simulink model "HANcoder_E407_GTSync_v3_clean"  (R2018b)
settings: Solver=FixedStepDiscrete  StartTime=0.0  StopTime=1  FixedStep=0.01  RelTol=1e-3
PreLoadFcn:
  | librarySetup
  | eval([bdroot,'_startup']) %Calling [modelName]_startup.m
values from neighbouring files (symbols this model uses):
  basic_cycle_duration = 60000    [HANcoder_E407_GTSync_v3_clean_startup.m]    (also in HANcoder_E407_GTSync_v3_startup.m = 50000)
  comm_delay_estimation = 3    [HANcoder_E407_GTSync_v3_clean_startup.m]
  frequency_IRQ = 100    [HANcoder_E407_GTSync_startup.m]    (also in HANcoder_E407_GTSync_v3_clean_startup.m = 99; HANcoder_E407_GTSync_v3_startup.m = 99)
  HANtuneOverride = Simulink.Parameter    [HANcoder_E407_GTSync_startup.m]    (also in HANcoder_E407_GTSync_v3_clean_startup.m; HANcoder_E407_GTSync_v3_startup.m)
  LED_ticks_toggle = 10000    [HANcoder_E407_GTSync_startup.m]    (also in HANcoder_E407_GTSync_v3_clean_startup.m; HANcoder_E407_GTSync_v3_startup.m)
  Master_Role = 1    [HANcoder_E407_GTSync_v3_clean_startup.m]    (also in HANcoder_E407_GTSync_v3_startup.m)
  matrix_rows = 2    [HANcoder_E407_GTSync_v3_clean_startup.m]    (also in HANcoder_E407_GTSync_v3_startup.m)
  Slave_Role = 2    [HANcoder_E407_GTSync_v3_clean_startup.m]    (also in HANcoder_E407_GTSync_v3_startup.m)
  Sync_ID = 1    [HANcoder_E407_GTSync_v3_clean_startup.m]    (also in HANcoder_E407_GTSync_v3_startup.m)
  time_difference_threshold = 500    [HANcoder_E407_GTSync_v3_clean_startup.m]    (also in HANcoder_E407_GTSync_v3_startup.m = 100)
  TM0 = 100    [HANcoder_E407_GTSync_v3_clean_startup.m]    (also in HANcoder_E407_GTSync_v3_startup.m = 0)
  TM1 = 20000    [HANcoder_E407_GTSync_v3_clean_startup.m]    (also in HANcoder_E407_GTSync_v3_startup.m = 25000)
  TM2 = 30000    [HANcoder_E407_GTSync_v3_clean_startup.m]    (also in HANcoder_E407_GTSync_v3_startup.m = 37500)
  TM3 = 40000    [HANcoder_E407_GTSync_v3_clean_startup.m]    (also in HANcoder_E407_GTSync_v3_startup.m)
  TM4 = 50000    [HANcoder_E407_GTSync_v3_clean_startup.m]
  Vote1_ID = 12    [HANcoder_E407_GTSync_v3_clean_startup.m]    (also in HANcoder_E407_GTSync_v3_startup.m)
  Vote2_ID = 22    [HANcoder_E407_GTSync_v3_clean_startup.m]    (also in HANcoder_E407_GTSync_v3_startup.m)
  Vote3_ID = 32    [HANcoder_E407_GTSync_v3_clean_startup.m]    (also in HANcoder_E407_GTSync_v3_startup.m)
  wrap_up_threshold = basic_cycle_duration - time_difference_threshold*10    (= 55000)    [HANcoder_E407_GTSync_v3_clean_startup.m]
libraries: HANcoder_STM32_Target x20, simulink x3, simulink_extras x1
(part 2 of 4)

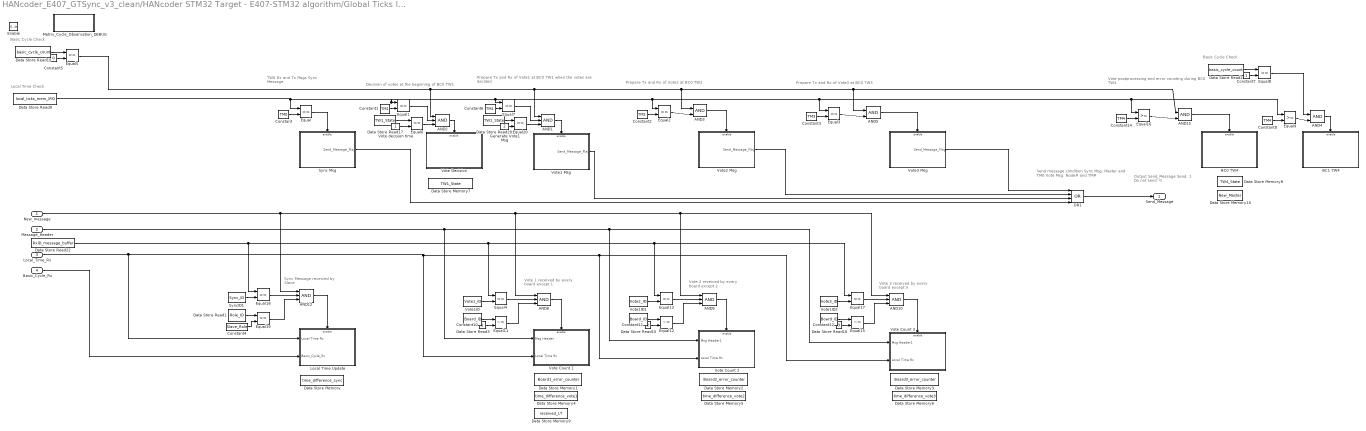
== system HANcoder_E407_GTSync_v3_clean/HANcoder STM32 Target - E407-STM32 algorithm/Global Ticks Increment/CAN Management/Matrix Cycle Manager ==
  note: Vote 3 received by
      | every board except 3
  note: Vote 2 received by
      | every board except 2
  note: Vote 1 received by
      | every board except 1
  note: Vote postprocessing and error
      | counting during BC0 TW4
  note: Prepare Tx and Rx of Vote3 at BC0 TW3
  note: Prepare Tx and Rx of Vote2 at BC0 TW2
  note: Prepare Tx and Rx of Vote1 at BC0 TW1
      | when the votes are decided
  note: Decision of votes at the beginning of BC0 TW1
  note: TW0 Rx and Tx Msgs
      | Sync Message
  note: Sync Message
      | received by Slave
  note: Local Time Check
  note: Output Send_Message
      | Send: 1
      | Do not send: 0
  note: Send message condition
      | Sync Msg: Master and TM0
      | Vote Msg: Node# and TM#
  note: Basic Cycle Check
  note: Basic Cycle Check
  New_message : Inport
  Message_Header : Inport  Port=2
  Local_Time_Rx : Inport  Port=3
  Basic_Cycle_Rx : Inport  Port=4
  Enable : EnablePort  PropagateVarSize=During execution
  AND{1..2,8..10,12} (6 alike) : Logic  Inputs=3  IconShape=distinctive  AllPortsSameDT=off  OutDataTypeStr=boolean
  AND{3..5,15} (4 alike) : Logic  IconShape=distinctive  AllPortsSameDT=off  OutDataTypeStr=boolean
  BC0 TW4 : Subsystem
  BC1 TW4 : Subsystem
  Constant : Constant  Value=TM0
  Constant1 : Constant  Value=TM1
  Constant10 : Constant
  Constant11 : Constant  Value=2
  Constant12 : Constant  Value=3
  Constant14 : Constant  Value=TM4
  Constant2 : Constant  Value=TM2
  Constant3 : Constant  Value=TM3
  Constant4 : Constant  Value=Slave_Role
  Constant5 : Constant  Value=0
  Constant6 : Constant  Value=TM1
  Constant7 : Constant
  Constant8 : Constant  Value=TM4
  Data Store Memory : DataStoreMemory  DataStoreName=time_difference_sync  ReadBeforeWriteMsg=warning  WriteAfterWriteMsg=warning  WriteAfterReadMsg=warning  ShowAdditionalParam=off
  Data Store Memory1 : DataStoreMemory  DataStoreName=Board1_error_counter  ReadBeforeWriteMsg=warning  WriteAfterWriteMsg=warning  WriteAfterReadMsg=warning  ShowAdditionalParam=off  OutMin=0  OutMax=4294967294  OutDataTypeStr=double
  Data Store Memory10 : DataStoreMemory  DataStoreName=New_Master  ReadBeforeWriteMsg=warning  WriteAfterWriteMsg=warning  WriteAfterReadMsg=warning  ShowAdditionalParam=off  OutDataTypeStr=boolean
  Data Store Memory2 : DataStoreMemory  DataStoreName=Board2_error_counter  ReadBeforeWriteMsg=warning  WriteAfterWriteMsg=warning  WriteAfterReadMsg=warning  ShowAdditionalParam=off  OutMin=0  OutMax=4294967294  OutDataTypeStr=double
  Data Store Memory3 : DataStoreMemory  DataStoreName=Board3_error_counter  ReadBeforeWriteMsg=warning  WriteAfterWriteMsg=warning  WriteAfterReadMsg=warning  ShowAdditionalParam=off  OutMin=0  OutMax=4294967294  OutDataTypeStr=double
  Data Store Memory4 : DataStoreMemory  DataStoreName=time_difference_vote1  ReadBeforeWriteMsg=warning  WriteAfterWriteMsg=warning  WriteAfterReadMsg=warning  ShowAdditionalParam=off
  Data Store Memory5 : DataStoreMemory  DataStoreName=time_difference_vote2  ReadBeforeWriteMsg=warning  WriteAfterWriteMsg=warning  WriteAfterReadMsg=warning  ShowAdditionalParam=off
  Data Store Memory6 : DataStoreMemory  DataStoreName=time_difference_vote3  ReadBeforeWriteMsg=warning  WriteAfterWriteMsg=warning  WriteAfterReadMsg=warning  ShowAdditionalParam=off
  Data Store Memory7 : DataStoreMemory  DataStoreName=TW1_State  ReadBeforeWriteMsg=warning  WriteAfterWriteMsg=warning  WriteAfterReadMsg=warning  InitialValue=1  ShowAdditionalParam=off
  Data Store Memory8 : DataStoreMemory  DataStoreName=TW4_State  ReadBeforeWriteMsg=warning  WriteAfterWriteMsg=warning  WriteAfterReadMsg=warning  InitialValue=1  ShowAdditionalParam=off
  Data Store Memory9 : DataStoreMemory  DataStoreName=received_LT  ReadBeforeWriteMsg=warning  WriteAfterWriteMsg=warning  WriteAfterReadMsg=warning  ShowAdditionalParam=off  OutDataTypeStr=Bus: received_vote_local_time
  Data Store Read1 : DataStoreRead  DataStoreName=Role_ID
  Data Store Read10 : DataStoreRead  DataStoreName=basic_cycle_count
  Data Store Read15 : DataStoreRead  DataStoreName=Board_ID
  Data Store Read16 : DataStoreRead  DataStoreName=Board_ID
  Data Store Read17 : DataStoreRead  DataStoreName=TW1_State
  Data Store Read2 : DataStoreRead  DataStoreName=basic_cycle_count
  Data Store Read20 : DataStoreRead  DataStoreName=TW1_State
  Data Store Read22 : DataStoreRead  DataStoreName=RxID_message_buffer
  Data Store Read3 : DataStoreRead  DataStoreName=Board_ID
  Data Store Read9 : DataStoreRead  DataStoreName=local_ticks_mem_IRQ
  Equal{,1..8,13,17..20} (14 alike) : RelationalOperator  Operator===  OutDataTypeStr=boolean  RndMeth=Simplest
  Equal11 : RelationalOperator  Operator=~=  OutDataTypeStr=boolean  RndMeth=Simplest
  Equal12 : RelationalOperator  Operator=~=  OutDataTypeStr=boolean  RndMeth=Simplest
  Equal15 : RelationalOperator  Operator=~=  OutDataTypeStr=boolean  RndMeth=Simplest
  Equal16 : RelationalOperator  OutDataTypeStr=boolean  RndMeth=Simplest
  Equal9 : RelationalOperator  OutDataTypeStr=boolean  RndMeth=Simplest
  Generate Vote1 Msg : Constant  Value=2
  Local Time Update : Subsystem
  Matrix_Cycle_Observation_DEBUG : Subsystem
  OR1 : Logic  Operator=OR  Inputs=4  IconShape=distinctive  AllPortsSameDT=off  OutDataTypeStr=boolean
  Sync Msg : Subsystem
  SyncID1 : Constant  Value=Sync_ID
  Vote Count 1 : Subsystem
  Vote Count 2 : Subsystem
  Vote Count 3 : Subsystem
  Vote Decision : Subsystem
  Vote decision time : Constant
  Vote1 Msg : Subsystem
  Vote1ID : Constant  Value=Vote1_ID
  Vote1ID1 : Constant  Value=Vote2_ID
  Vote1ID2 : Constant  Value=Vote3_ID
  Vote2 Msg : Subsystem
  Vote3 Msg : Subsystem
  Send_Message : Outport
  wires:
  Constant3/1 -> Equal3/2
  Data Store Read10/1 -> Equal5/1
  Constant5/1 -> Equal5/2
  Constant/1 -> Equal/2
  Constant2/1 -> Equal2/2
  Equal3/1 -> AND5/2
  Constant1/1 -> Equal1/2
  Equal1/1 -> AND2/2
  Equal2/1 -> AND3/2
  OR1/1 -> Send_Message/1
  Equal/1 -> Sync Msg/Enable
  Equal16/1 -> AND15/2
  Constant14/1 -> Equal16/2
  AND3/1 -> Vote2 Msg/Enable
  AND5/1 -> Vote3 Msg/Enable
  Sync Msg/1(Send_Message_Flag) -> OR1/4
  Vote1 Msg/1(Send_Message_Flag) -> OR1/3
  Vote2 Msg/1(Send_Message_Flag) -> OR1/2
  Vote3 Msg/1(Send_Message_Flag) -> OR1/1
  AND15/1 -> BC0 TW4/Enable
  Local_Time_Rx/1 -> Local Time Update/1(Local Time Rx), Vote Count 2/2(Local Time Rx), Vote Count 3/2(Local Time Rx), Vote Count 1/2(Local Time Rx)
  AND12/1 -> Local Time Update/Enable
  SyncID1/1 -> Equal18/2
  Equal18/1 -> AND12/2
  Data Store Read1/1 -> Equal19/1
  Constant4/1 -> Equal19/2
  Equal19/1 -> AND12/3
  Vote1ID/1 -> Equal4/2
  Equal4/1 -> AND8/2
  Equal11/1 -> AND8/3
  Constant10/1 -> Equal11/2
  Data Store Read3/1 -> Equal11/1
  AND8/1 -> Vote Count 1/Enable
  AND9/1 -> Vote Count 2/Enable
  Data Store Read15/1 -> Equal12/1
  Constant11/1 -> Equal12/2
  Equal12/1 -> AND9/3
  Equal13/1 -> AND9/2
  Vote1ID1/1 -> Equal13/2
  Data Store Read22/1 -> Equal18/1, Equal4/1, Equal13/1, Equal17/1
  New_message/1 -> AND12/1, AND8/1, AND9/1, AND10/1
  Message_Header/1 -> Vote Count 1/1(Msg Header), Vote Count 3/1(Msg Header1), Vote Count 2/1(Msg Header1)
  Vote1ID2/1 -> Equal17/2
  Equal17/1 -> AND10/2
  Equal15/1 -> AND10/3
  Constant12/1 -> Equal15/2
  Data Store Read16/1 -> Equal15/1
  AND10/1 -> Vote Count 3/Enable
  Vote decision time/1 -> Equal6/2
  AND2/1 -> Vote Decision/Enable
  Data Store Read17/1 -> Equal6/1
  Data Store Read20/1 -> Equal20/1
  Generate Vote1 Msg/1 -> Equal20/2
  Equal20/1 -> AND1/3
  Equal6/1 -> AND2/3
  Basic_Cycle_Rx/1 -> Local Time Update/2(Basic_Cycle_Rx)
  Equal5/1 -> AND15/1, AND5/1, AND3/1, AND1/1, AND2/1
  Equal7/1 -> AND1/2
  Constant6/1 -> Equal7/2
  AND1/1 -> Vote1 Msg/Enable
  Equal8/1 -> AND4/1
  Constant7/1 -> Equal8/2
  Data Store Read2/1 -> Equal8/1
  Data Store Read9/1 -> Equal1/1, Equal7/1, Equal9/1, Equal16/1, Equal3/1, Equal2/1, Equal/1
  Constant8/1 -> Equal9/2
  Equal9/1 -> AND4/2
  AND4/1 -> BC1 TW4/Enable

== system HANcoder_E407_GTSync_v3_clean/HANcoder STM32 Target - E407-STM32 algorithm/Global Ticks Increment/Send/CAN send ==
  In1 : Inport
  In2 : Inport  Port=2
  In3 : Inport  Port=3
  In4 : Inport  Port=4
  In5 : Inport  Port=5
  In6 : Inport  Port=6
  In7 : Inport  Port=7
  In8 : Inport  Port=8
  In9 : Inport  Port=9
  S-Function : M-S-Function  FunctionName=sfcn_can_send  Parameters=tsamp, canBus, frameType, inputNumber, dataType, byteOrder
  wires:
  In1/1 -> S-Function/1
  In2/1 -> S-Function/2
  In3/1 -> S-Function/3
  In4/1 -> S-Function/4
  In5/1 -> S-Function/5
  In6/1 -> S-Function/6
  In7/1 -> S-Function/7
  In8/1 -> S-Function/8
  In9/1 -> S-Function/9

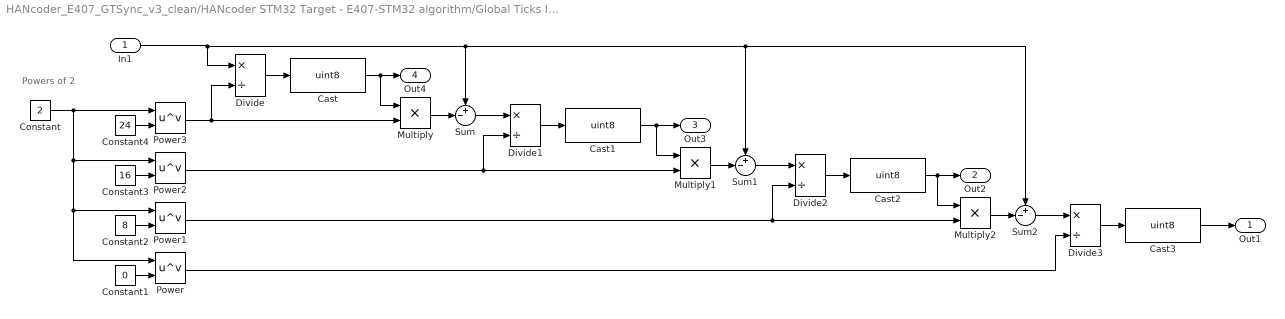
== system HANcoder_E407_GTSync_v3_clean/HANcoder STM32 Target - E407-STM32 algorithm/Global Ticks Increment/Send/UINT32 to UINT8 ==
  note: Powers of 2
  In1 : Inport
  Cast{,1..3} (4 alike) : DataTypeConversion  OutDataTypeStr=uint8
  Constant : Constant  Value=2
  Constant1 : Constant  Value=0
  Constant2 : Constant  Value=8
  Constant3 : Constant  Value=16
  Constant4 : Constant  Value=24
  Divide{,1..3} (4 alike) : Product  Inputs=*/
  Multiply : Product
  Multiply1 : Product
  Multiply2 : Product
  Power{,1..3} (4 alike) : Math  Operator=pow  SaturateOnIntegerOverflow=on
  Sum : Sum  Inputs=+-|
  Sum1 : Sum  Inputs=+-|
  Sum2 : Sum  Inputs=+-|
  Out1 : Outport
  Out2 : Outport  Port=2
  Out3 : Outport  Port=3
  Out4 : Outport  Port=4
  wires:
  Constant2/1 -> Power1/2
  Constant3/1 -> Power2/2
  Constant4/1 -> Power3/2
  Power2/1 -> Multiply1/2, Divide1/2
  Constant1/1 -> Power/2
  Power3/1 -> Divide/2, Multiply/2
  Constant/1 -> Power/1, Power1/1, Power2/1, Power3/1
  Divide/1 -> Cast/1
  Cast/1 -> Multiply/1, Out4/1
  Multiply/1 -> Sum/2
  Divide1/1 -> Cast1/1
  Sum/1 -> Divide1/1
  Cast1/1 -> Out3/1, Multiply1/1
  Multiply1/1 -> Sum1/2
  Multiply2/1 -> Sum2/2
  Cast2/1 -> Out2/1, Multiply2/1
  Divide2/1 -> Cast2/1
  Power1/1 -> Multiply2/2, Divide2/2
  Sum1/1 -> Divide2/1
  Sum2/1 -> Divide3/1
  In1/1 -> Sum1/1, Sum2/1, Sum/1, Divide/1
  Power/1 -> Divide3/2
  Divide3/1 -> Cast3/1
  Cast3/1 -> Out1/1

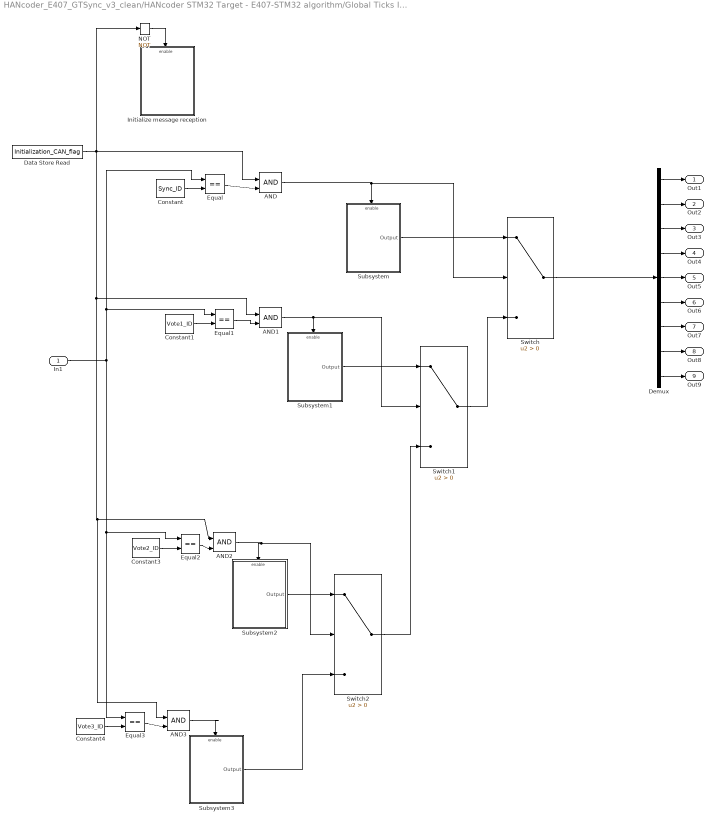
== system HANcoder_E407_GTSync_v3_clean/HANcoder STM32 Target - E407-STM32 algorithm/Global Ticks Increment/CAN Management/CAN Recieve/CAN Receive System ==
  In1 : Inport
  AND{,1..3} (4 alike) : Logic  IconShape=distinctive  AllPortsSameDT=off  OutDataTypeStr=boolean
  Constant : Constant  Value=Sync_ID  OutDataTypeStr=uint32
  Constant1 : Constant  Value=Vote1_ID  OutDataTypeStr=uint32
  Constant3 : Constant  Value=Vote2_ID  OutDataTypeStr=uint32
  Constant4 : Constant  Value=Vote3_ID  OutDataTypeStr=uint32
  Data Store Read : DataStoreRead  DataStoreName=Initialization_CAN_flag
  Demux : Demux  Outputs=9
  Equal{,1..3} (4 alike) : RelationalOperator  Operator===  OutDataTypeStr=boolean  RndMeth=Simplest
  Initialize message reception : Subsystem
  NOT : Logic  Operator=NOT  IconShape=distinctive  AllPortsSameDT=off  OutDataTypeStr=boolean
  Subsystem : Subsystem
  Subsystem1 : Subsystem
  Subsystem2 : Subsystem
  Subsystem3 : Subsystem
  Switch : Switch  Criteria=u2 > Threshold
  Switch1 : Switch  Criteria=u2 > Threshold
  Switch2 : Switch  Criteria=u2 > Threshold
  Out1 : Outport
  Out2 : Outport  Port=2
  Out3 : Outport  Port=3
  Out4 : Outport  Port=4
  Out5 : Outport  Port=5
  Out6 : Outport  Port=6
  Out7 : Outport  Port=7
  Out8 : Outport  Port=8
  Out9 : Outport  Port=9
  wires:
  Demux/1 -> Out1/1
  Demux/2 -> Out2/1
  Demux/3 -> Out3/1
  Demux/4 -> Out4/1
  Demux/5 -> Out5/1
  Demux/6 -> Out6/1
  Demux/7 -> Out7/1
  Demux/8 -> Out8/1
  Demux/9 -> Out9/1
  Switch/1 -> Demux/1
  Constant/1 -> Equal/2
  Equal/1 -> AND/2
  Constant1/1 -> Equal1/2
  Constant3/1 -> Equal2/2
  Constant4/1 -> Equal3/2
  In1/1 -> Equal1/1, Equal/1, Equal3/1, Equal2/1
  Equal1/1 -> AND1/2
  Equal2/1 -> AND2/2
  Equal3/1 -> AND3/2
  Subsystem/1(Output) -> Switch/1
  Switch1/1 -> Switch/3
  Subsystem1/1(Output) -> Switch1/1
  Subsystem3/1(Output) -> Switch2/3
  Switch2/1 -> Switch1/3
  Subsystem2/1(Output) -> Switch2/1
  AND/1 -> Switch/2, Subsystem/Enable
  Data Store Read/1 -> NOT/1, AND/1, AND3/1, AND2/1, AND1/1
  AND1/1 -> Switch1/2, Subsystem1/Enable
  AND2/1 -> Switch2/2, Subsystem2/Enable
  AND3/1 -> Subsystem3/Enable
  NOT/1 -> Initialize message reception/Enable

== system HANcoder_E407_GTSync_v3_clean/HANcoder STM32 Target - E407-STM32 algorithm/Global Ticks Increment/CAN Management/CAN Recieve/UINT8 to UINT32 ==
  note: Each uint8 is multiplied by the power of 2 corresponding to its position in the uint32 output
  note: Powers of 2
  In1 : Inport
  In2 : Inport  Port=2
  In3 : Inport  Port=3
  In4 : Inport  Port=4
  Cast : DataTypeConversion  OutDataTypeStr=uint32
  Constant : Constant  Value=2
  Constant1 : Constant  Value=0
  Constant2 : Constant  Value=8
  Constant3 : Constant  Value=16
  Constant4 : Constant  Value=24
  Multiply{,1..3} (4 alike) : Product
  Power{,1..3} (4 alike) : Math  Operator=pow  SaturateOnIntegerOverflow=on
  Sum : Sum  Inputs=++++
  Out1 : Outport
  wires:
  Cast/1 -> Out1/1
  Sum/1 -> Cast/1
  In1/1 -> Multiply1/1
  In2/1 -> Multiply/1
  In3/1 -> Multiply2/1
  In4/1 -> Multiply3/1
  Constant/1 -> Power3/1, Power2/1, Power1/1, Power/1
  Constant1/1 -> Power/2
  Constant2/1 -> Power1/2
  Constant3/1 -> Power2/2
  Constant4/1 -> Power3/2
  Power/1 -> Multiply1/2
  Power1/1 -> Multiply/2
  Power2/1 -> Multiply2/2
  Power3/1 -> Multiply3/2
  Multiply3/1 -> Sum/4
  Multiply2/1 -> Sum/3
  Multiply/1 -> Sum/2
  Multiply1/1 -> Sum/1

== system HANcoder_E407_GTSync_v3_clean/HANcoder STM32 Target - E407-STM32 algorithm/Global Ticks Increment/CAN Management/Matrix Cycle Manager/BC0 TW4 ==
  note: Basic Cycle 0
      | Time Window 4
      | 	No message communication
      | 	1 - Previous message timeouts ( _processed variables )
      | 	2 - MasterID decision
      | 	3 - Variables reset
  Enable : EnablePort  PropagateVarSize=During execution
  Data Store Read : DataStoreRead  DataStoreName=TW4_State
  Data Store Read2 : DataStoreRead  DataStoreName=TW4_State
  Data Store Read3 : DataStoreRead  DataStoreName=TW4_State
  Equal : RelationalOperator  Operator===  OutDataTypeStr=boolean  RndMeth=Simplest
  Equal2 : RelationalOperator  Operator===  OutDataTypeStr=boolean  RndMeth=Simplest
  Equal3 : RelationalOperator  Operator===  OutDataTypeStr=boolean  RndMeth=Simplest
  Master ID decision : Constant  Value=2
  Reset variables : Constant  Value=3
  Subsystem : Subsystem
  Subsystem2 : Subsystem
  Subsystem3 : Subsystem
  Timeouts Check : Constant
  wires:
  Data Store Read/1 -> Equal/1
  Timeouts Check/1 -> Equal/2
  Equal/1 -> Subsystem/Enable
  Data Store Read2/1 -> Equal2/1
  Master ID decision/1 -> Equal2/2
  Equal2/1 -> Subsystem2/Enable
  Equal3/1 -> Subsystem3/Enable
  Reset variables/1 -> Equal3/2
  Data Store Read3/1 -> Equal3/1

== system HANcoder_E407_GTSync_v3_clean/HANcoder STM32 Target - E407-STM32 algorithm/Global Ticks Increment/CAN Management/Matrix Cycle Manager/BC1 TW4 ==
  note: Basic Cycle 1
      | Time Window 4
      | 	No message communication
      | 	1 - Variables reset
  Enable : EnablePort  PropagateVarSize=During execution
  Data Store Read3 : DataStoreRead  DataStoreName=TW4_State
  Equal3 : RelationalOperator  Operator===  OutDataTypeStr=boolean  RndMeth=Simplest
  Reset variables : Constant  Value=4
  Subsystem3 : Subsystem
  wires:
  Data Store Read3/1 -> Equal3/1
  Reset variables/1 -> Equal3/2
  Equal3/1 -> Subsystem3/Enable

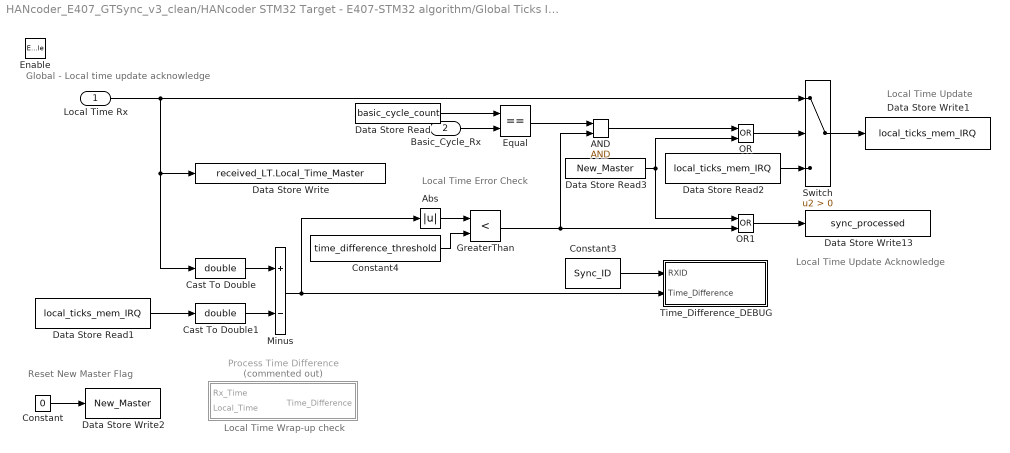
== system HANcoder_E407_GTSync_v3_clean/HANcoder STM32 Target - E407-STM32 algorithm/Global Ticks Increment/CAN Management/Matrix Cycle Manager/Local Time Update ==
  note: Reset New Master Flag
  note: Local Time Wrap-up check
  note: Local Time Error Check
  note: Local Time Update
  note: Local Time Update Acknowledge
  note: Global - Local time update acknowledge
  Local Time Rx : Inport
  Basic_Cycle_Rx : Inport  Port=2
  Enable : EnablePort
  AND : Logic  IconShape=distinctive  AllPortsSameDT=off  OutDataTypeStr=boolean
  Abs : Abs
  Cast To Double : DataTypeConversion  OutDataTypeStr=double
  Cast To Double1 : DataTypeConversion  OutDataTypeStr=double
  Constant : Constant  Value=0  OutDataTypeStr=boolean
  Constant3 : Constant  Value=Sync_ID
  Constant4 : Constant  Value=time_difference_threshold
  Data Store Read : DataStoreRead  DataStoreName=basic_cycle_count
  Data Store Read1 : DataStoreRead  DataStoreName=local_ticks_mem_IRQ
  Data Store Read2 : DataStoreRead  DataStoreName=local_ticks_mem_IRQ
  Data Store Read3 : DataStoreRead  DataStoreName=New_Master
  Data Store Write : DataStoreWrite  DataStoreName=received_LT  DataStoreElements=received_LT.Local_Time_Master
  Data Store Write1 : DataStoreWrite  DataStoreName=local_ticks_mem_IRQ
  Data Store Write13 : DataStoreWrite  DataStoreName=sync_processed
  Data Store Write2 : DataStoreWrite  DataStoreName=New_Master
  Equal : RelationalOperator  Operator===  OutDataTypeStr=boolean  RndMeth=Simplest
  GreaterThan : RelationalOperator  Operator=<  OutDataTypeStr=boolean  RndMeth=Simplest
  Minus : Sum  Inputs=+-
  OR : Logic  Operator=OR  IconShape=distinctive  AllPortsSameDT=off  OutDataTypeStr=boolean
  OR1 : Logic  Operator=OR  IconShape=distinctive  AllPortsSameDT=off  OutDataTypeStr=boolean
  Process Time Difference : Subsystem  Commented=on
  Switch : Switch  Criteria=u2 > Threshold
  Time_Difference_DEBUG : Subsystem
  wires:
  Constant3/1 -> Time_Difference_DEBUG/1(RXID)
  Minus/1 -> Time_Difference_DEBUG/2(Time_Difference), Abs/1
  Abs/1 -> GreaterThan/1
  Constant4/1 -> GreaterThan/2
  GreaterThan/1 -> AND/2, OR1/2
  Data Store Read1/1 -> Cast To Double1/1
  Data Store Read2/1 -> Switch/3
  Local Time Rx/1 -> Data Store Write/1, Cast To Double/1, Switch/1
  Switch/1 -> Data Store Write1/1
  AND/1 -> OR/1
  Data Store Read/1 -> Equal/1
  Equal/1 -> AND/1
  Basic_Cycle_Rx/1 -> Equal/2
  Cast To Double/1 -> Minus/1
  Cast To Double1/1 -> Minus/2
  Data Store Read3/1 -> OR/2, OR1/1
  OR/1 -> Switch/2
  OR1/1 -> Data Store Write13/1
  Constant/1 -> Data Store Write2/1

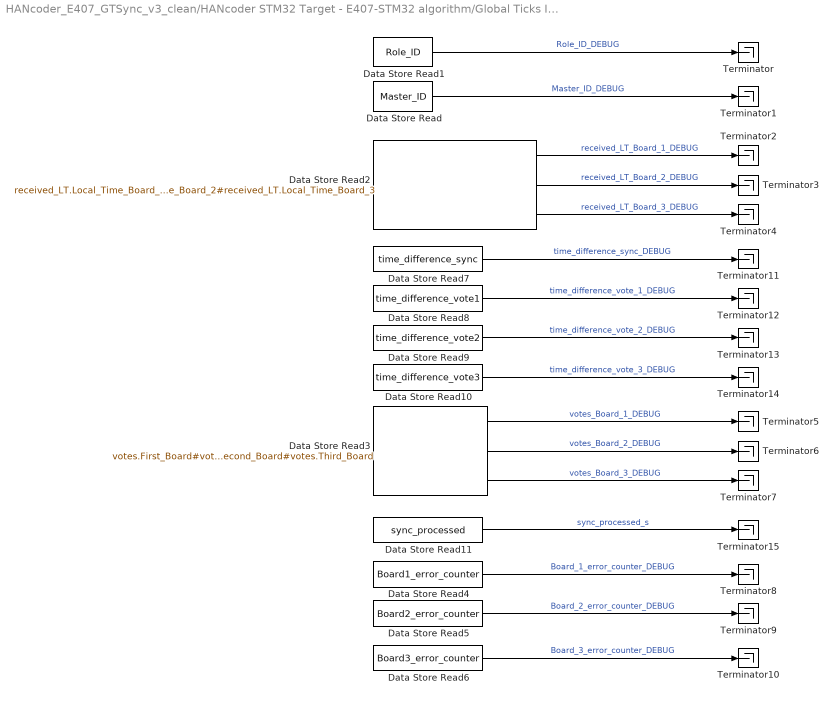
== system HANcoder_E407_GTSync_v3_clean/HANcoder STM32 Target - E407-STM32 algorithm/Global Ticks Increment/CAN Management/Matrix Cycle Manager/Matrix_Cycle_Observation_DEBUG ==
  Data Store Read : DataStoreRead  DataStoreName=Master_ID
  Data Store Read1 : DataStoreRead  DataStoreName=Role_ID
  Data Store Read10 : DataStoreRead  DataStoreName=time_difference_vote3
  Data Store Read11 : DataStoreRead  DataStoreName=sync_processed
  Data Store Read2 : DataStoreRead  DataStoreName=received_LT  DataStoreElements=received_LT.Local_Time_Board_1#received_LT.Local_Time_Board_2#received_LT.Local_Time_Board_3
  Data Store Read3 : DataStoreRead  DataStoreName=votes  DataStoreElements=votes.First_Board#votes.Second_Board#votes.Third_Board
  Data Store Read4 : DataStoreRead  DataStoreName=Board1_error_counter
  Data Store Read5 : DataStoreRead  DataStoreName=Board2_error_counter
  Data Store Read6 : DataStoreRead  DataStoreName=Board3_error_counter
  Data Store Read7 : DataStoreRead  DataStoreName=time_difference_sync
  Data Store Read8 : DataStoreRead  DataStoreName=time_difference_vote1
  Data Store Read9 : DataStoreRead  DataStoreName=time_difference_vote2
  Terminator{,1..15} (16 alike) : Terminator
  wires:
  Data Store Read1/1 -> Terminator/1  "Role_ID_DEBUG"
  Data Store Read/1 -> Terminator1/1  "Master_ID_DEBUG"
  Data Store Read2/1 -> Terminator2/1  "received_LT_Board_1_DEBUG"
  Data Store Read2/2 -> Terminator3/1  "received_LT_Board_2_DEBUG"
  Data Store Read2/3 -> Terminator4/1  "received_LT_Board_3_DEBUG"
  Data Store Read3/1 -> Terminator5/1  "votes_Board_1_DEBUG"
  Data Store Read3/2 -> Terminator6/1  "votes_Board_2_DEBUG"
  Data Store Read3/3 -> Terminator7/1  "votes_Board_3_DEBUG"
  Data Store Read4/1 -> Terminator8/1  "Board_1_error_counter_DEBUG"
  Data Store Read5/1 -> Terminator9/1  "Board_2_error_counter_DEBUG"
  Data Store Read6/1 -> Terminator10/1  "Board_3_error_counter_DEBUG"
  Data Store Read7/1 -> Terminator11/1  "time_difference_sync_DEBUG"
  Data Store Read8/1 -> Terminator12/1  "time_difference_vote_1_DEBUG"
  Data Store Read9/1 -> Terminator13/1  "time_difference_vote_2_DEBUG"
  Data Store Read10/1 -> Terminator14/1  "time_difference_vote_3_DEBUG"
  Data Store Read11/1 -> Terminator15/1  "sync_processed_s"

== system HANcoder_E407_GTSync_v3_clean/HANcoder STM32 Target - E407-STM32 algorithm/Global Ticks Increment/CAN Management/Matrix Cycle Manager/Sync Msg ==
  note: Message Data (2)
      |    Basic cycle for Sync
  note: Send Message condition
  note: Basic Cycle 0
      | Time Window 0
      | Message Sent: < Only if RoleID == 1 (Master) >
      | 	TxMessage ID: Sync
      | 	Message Header: BoardID
      | 	Message buffert : Local Time
      | Message Receive: < Only if RoleID ~= 1 (Slave)>
      | 	RxMessage ID: Sync
  note: Message Data
      |    Every message sends
      |    Local_Time as Data
  note: Transmission ID
      |    Sync Msg: 1
      |    Vote Node 1: 12
      |    Vote Node 2: 22
      |    Vote Node 3: 32
  note: Message Information
      |    Sync: BoardID
      |    Vote: Vote information
  note: Reception ID
      |    Sync Msg: 1
      |    Vote Node 1: 12
      |    Vote Node 2: 22
      |    Vote Node 3: 32
  Enable : EnablePort
  Cast : DataTypeConversion  OutDataTypeStr=uint32
  Cast1 : DataTypeConversion  OutDataTypeStr=uint32
  Cast2 : DataTypeConversion  OutDataTypeStr=uint8
  Cast3 : DataTypeConversion  OutDataTypeStr=uint32
  Cast4 : DataTypeConversion  OutDataTypeStr=uint8
  Constant : Constant  Value=Sync_ID
  Constant1 : Constant  Value=Master_Role
  Constant18 : Constant  Value=comm_delay_estimation
  Constant2 : Constant  Value=Sync_ID
  Data Store Read : DataStoreRead  DataStoreName=local_ticks_mem_IRQ
  Data Store Read1 : DataStoreRead  DataStoreName=Role_ID
  Data Store Read2 : DataStoreRead  DataStoreName=Board_ID
  Data Store Read3 : DataStoreRead  DataStoreName=basic_cycle_count
  Data Store Write1 : DataStoreWrite  DataStoreName=message_buffer_2
  Data Store Write5 : DataStoreWrite  DataStoreName=message_header_buffer
  Data Store Write6 : DataStoreWrite  DataStoreName=RxID_message_buffer
  Data Store Write8 : DataStoreWrite  DataStoreName=TxID_message_buffer
  Data Store Write9 : DataStoreWrite  DataStoreName=message_buffer
  Equal : RelationalOperator  Operator===  OutDataTypeStr=boolean  RndMeth=Simplest
  Minus1 : Sum
  Send_Message_Flag : Outport  OutputWhenDisabled=reset  InitialOutput=0
  wires:
  Constant18/1 -> Minus1/2
  Minus1/1 -> Cast1/1
  Cast1/1 -> Data Store Write9/1
  Cast/1 -> Data Store Write8/1
  Data Store Read/1 -> Minus1/1
  Constant/1 -> Cast/1
  Data Store Read1/1 -> Equal/1
  Equal/1 -> Send_Message_Flag/1
  Constant1/1 -> Equal/2
  Cast3/1 -> Data Store Write6/1
  Constant2/1 -> Cast3/1
  Cast2/1 -> Data Store Write5/1
  Cast4/1 -> Data Store Write1/1
  Data Store Read3/1 -> Cast4/1
  Data Store Read2/1 -> Cast2/1

== system HANcoder_E407_GTSync_v3_clean/HANcoder STM32 Target - E407-STM32 algorithm/Global Ticks Increment/CAN Management/Matrix Cycle Manager/Vote Count 1 ==
  note: Take vote into account if the board was synced
  note: Local Time Received Check
  note: Msg Received
  Msg Header : Inport
  Local Time Rx : Inport  Port=2
  Enable : EnablePort
  Abs : Abs
  Cast To Double : DataTypeConversion  OutDataTypeStr=double
  Cast To Double1 : DataTypeConversion  OutDataTypeStr=double
  Constant3 : Constant  Value=Vote1_ID
  Constant4 : Constant  Value=time_difference_threshold
  Constant6 : Constant
  Data Store Read : DataStoreRead  DataStoreName=Board1_error_counter
  Data Store Read1 : DataStoreRead  DataStoreName=local_ticks_mem_IRQ
  Data Store Read5 : DataStoreRead  DataStoreName=Board1_error_counter
  Data Store Write : DataStoreWrite  DataStoreName=BC0_TM1_processed
  Data Store Write1 : DataStoreWrite  DataStoreName=Board1_error_counter
  Data Store Write2 : DataStoreWrite  DataStoreName=received_LT  DataStoreElements=received_LT.Local_Time_Board_1
  GreaterThan : RelationalOperator  Operator=>  OutDataTypeStr=boolean  RndMeth=Simplest
  HIGH : Constant  OutDataTypeStr=boolean
  Minus : Sum  Inputs=+-
  NOT : Logic  Operator=NOT  IconShape=distinctive  AllPortsSameDT=off  OutDataTypeStr=boolean
  Plus : Sum
  Sum up new vote : Subsystem
  Switch2 : Switch  Criteria=u2 > Threshold
  Time_Difference_DEBUG : Subsystem
  wires:
  HIGH/1 -> Data Store Write/1
  Minus/1 -> Time_Difference_DEBUG/2(Time_Difference), Abs/1
  Constant3/1 -> Time_Difference_DEBUG/1(RXID)
  Data Store Read1/1 -> Cast To Double1/1
  Abs/1 -> GreaterThan/1
  Constant4/1 -> GreaterThan/2
  Data Store Read5/1 -> Plus/1
  Plus/1 -> Switch2/1
  Constant6/1 -> Plus/2
  GreaterThan/1 -> Switch2/2, NOT/1
  Data Store Read/1 -> Switch2/3
  Switch2/1 -> Data Store Write1/1
  Local Time Rx/1 -> Cast To Double/1, Data Store Write2/1
  Cast To Double/1 -> Minus/1
  Cast To Double1/1 -> Minus/2
  Msg Header/1 -> Sum up new vote/1(Msg Header)
  NOT/1 -> Sum up new vote/Enable

== system HANcoder_E407_GTSync_v3_clean/HANcoder STM32 Target - E407-STM32 algorithm/Global Ticks Increment/CAN Management/Matrix Cycle Manager/Vote Count 2 ==
  note: Msg Received
  note: Local Time Received Check
  note: Take vote into account if the board was synced
  Msg Header1 : Inport
  Local Time Rx : Inport  Port=2
  Enable : EnablePort
  Abs : Abs
  Cast To Double : DataTypeConversion  OutDataTypeStr=double
  Cast To Double1 : DataTypeConversion  OutDataTypeStr=double
  Constant3 : Constant  Value=Vote2_ID
  Constant4 : Constant  Value=time_difference_threshold
  Constant6 : Constant
  Data Store Read : DataStoreRead  DataStoreName=Board2_error_counter
  Data Store Read1 : DataStoreRead  DataStoreName=local_ticks_mem_IRQ
  Data Store Read5 : DataStoreRead  DataStoreName=Board2_error_counter
  Data Store Write : DataStoreWrite  DataStoreName=BC0_TM2_processed
  Data Store Write1 : DataStoreWrite  DataStoreName=Board2_error_counter
  Data Store Write2 : DataStoreWrite  DataStoreName=received_LT  DataStoreElements=received_LT.Local_Time_Board_2
  GreaterThan : RelationalOperator  Operator=>  OutDataTypeStr=boolean  RndMeth=Simplest
  HIGH : Constant  OutDataTypeStr=boolean
  Minus : Sum  Inputs=+-
  NOT : Logic  Operator=NOT  IconShape=distinctive  AllPortsSameDT=off  OutDataTypeStr=boolean
  Plus : Sum
  Sum up new vote : Subsystem
  Switch2 : Switch  Criteria=u2 > Threshold
  Time_Difference_DEBUG : Subsystem
  wires:
  Switch2/1 -> Data Store Write1/1
  Data Store Read/1 -> Switch2/3
  Constant6/1 -> Plus/2
  Plus/1 -> Switch2/1
  Data Store Read5/1 -> Plus/1
  Constant4/1 -> GreaterThan/2
  Abs/1 -> GreaterThan/1
  Data Store Read1/1 -> Cast To Double1/1
  Constant3/1 -> Time_Difference_DEBUG/1(RXID)
  Minus/1 -> Abs/1, Time_Difference_DEBUG/2(Time_Difference)
  HIGH/1 -> Data Store Write/1
  Local Time Rx/1 -> Data Store Write2/1, Cast To Double/1
  Cast To Double/1 -> Minus/1
  Cast To Double1/1 -> Minus/2
  GreaterThan/1 -> Switch2/2, NOT/1
  Msg Header1/1 -> Sum up new vote/1(Msg Header)
  NOT/1 -> Sum up new vote/Enable

== system HANcoder_E407_GTSync_v3_clean/HANcoder STM32 Target - E407-STM32 algorithm/Global Ticks Increment/CAN Management/Matrix Cycle Manager/Vote Count 3 ==
  note: Local Time Received Check
  note: Msg Received
  note: Take vote into account if the board was synced
  Msg Header1 : Inport
  Local Time Rx : Inport  Port=2
  Enable : EnablePort
  Abs : Abs
  Cast To Double : DataTypeConversion  OutDataTypeStr=double
  Cast To Double1 : DataTypeConversion  OutDataTypeStr=double
  Constant3 : Constant  Value=Vote3_ID
  Constant4 : Constant  Value=time_difference_threshold
  Constant6 : Constant
  Data Store Read : DataStoreRead  DataStoreName=Board3_error_counter
  Data Store Read1 : DataStoreRead  DataStoreName=local_ticks_mem_IRQ
  Data Store Read5 : DataStoreRead  DataStoreName=Board3_error_counter
  Data Store Write : DataStoreWrite  DataStoreName=BC0_TM3_processed
  Data Store Write1 : DataStoreWrite  DataStoreName=Board3_error_counter
  Data Store Write2 : DataStoreWrite  DataStoreName=received_LT  DataStoreElements=received_LT.Local_Time_Board_3
  GreaterThan : RelationalOperator  Operator=>  OutDataTypeStr=boolean  RndMeth=Simplest
  HIGH : Constant  OutDataTypeStr=boolean
  Minus : Sum  Inputs=+-
  NOT : Logic  Operator=NOT  IconShape=distinctive  AllPortsSameDT=off  OutDataTypeStr=boolean
  Plus : Sum
  Sum up new vote : Subsystem
  Switch2 : Switch  Criteria=u2 > Threshold
  Time_Difference_DEBUG : Subsystem
  wires:
  HIGH/1 -> Data Store Write/1
  Minus/1 -> Time_Difference_DEBUG/2(Time_Difference), Abs/1
  Constant3/1 -> Time_Difference_DEBUG/1(RXID)
  Data Store Read1/1 -> Cast To Double1/1
  Abs/1 -> GreaterThan/1
  Constant4/1 -> GreaterThan/2
  Data Store Read5/1 -> Plus/1
  Plus/1 -> Switch2/1
  Constant6/1 -> Plus/2
  Data Store Read/1 -> Switch2/3
  Switch2/1 -> Data Store Write1/1
  Local Time Rx/1 -> Data Store Write2/1, Cast To Double/1
  Cast To Double/1 -> Minus/1
  Cast To Double1/1 -> Minus/2
  GreaterThan/1 -> NOT/1, Switch2/2
  Msg Header1/1 -> Sum up new vote/1(Msg Header)
  NOT/1 -> Sum up new vote/Enable

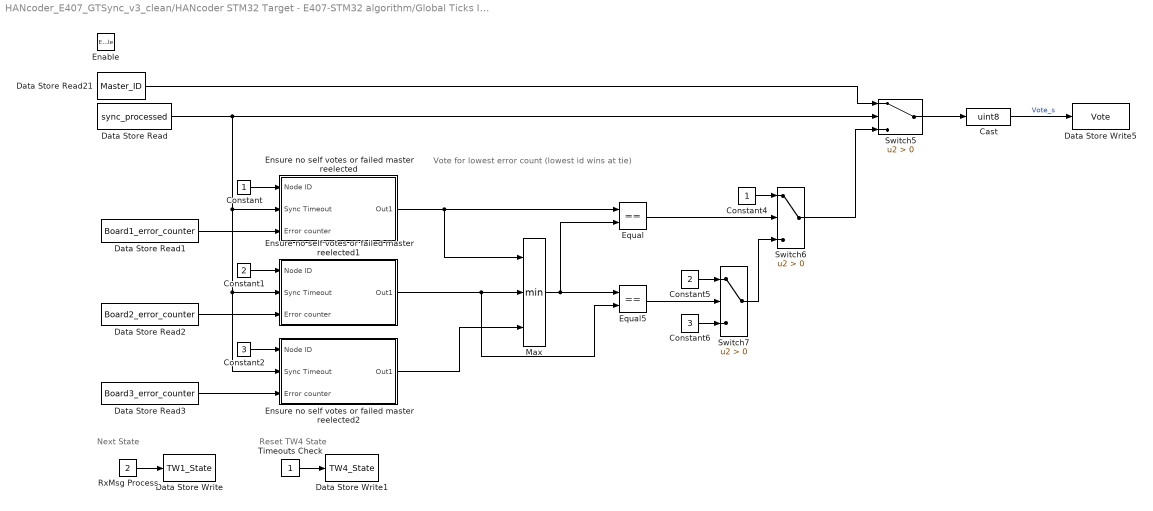
== system HANcoder_E407_GTSync_v3_clean/HANcoder STM32 Target - E407-STM32 algorithm/Global Ticks Increment/CAN Management/Matrix Cycle Manager/Vote Decision ==
  note: Next State
  note: Vote for lowest error count (lowest id wins at tie)
  note: Reset TW4 State
  Enable : EnablePort
  Cast : DataTypeConversion  OutDataTypeStr=uint8
  Constant : Constant
  Constant1 : Constant  Value=2
  Constant2 : Constant  Value=3
  Constant4 : Constant
  Constant5 : Constant  Value=2
  Constant6 : Constant  Value=3
  Data Store Read : DataStoreRead  DataStoreName=sync_processed
  Data Store Read1 : DataStoreRead  DataStoreName=Board1_error_counter
  Data Store Read2 : DataStoreRead  DataStoreName=Board2_error_counter
  Data Store Read21 : DataStoreRead  DataStoreName=Master_ID
  Data Store Read3 : DataStoreRead  DataStoreName=Board3_error_counter
  Data Store Write : DataStoreWrite  DataStoreName=TW1_State
  Data Store Write1 : DataStoreWrite  DataStoreName=TW4_State
  Data Store Write5 : DataStoreWrite  DataStoreName=Vote
  Ensure no self votes or failed master reelected : Subsystem
  Ensure no self votes or failed master reelected1 : Subsystem
  Ensure no self votes or failed master reelected2 : Subsystem
  Equal : RelationalOperator  Operator===  OutDataTypeStr=boolean  RndMeth=Simplest
  Equal5 : RelationalOperator  Operator===  OutDataTypeStr=boolean  RndMeth=Simplest
  Max : MinMax  Inputs=3
  RxMsg Process : Constant  Value=2
  Switch5 : Switch  Criteria=u2 > Threshold
  Switch6 : Switch  Criteria=u2 > Threshold
  Switch7 : Switch  Criteria=u2 > Threshold
  Timeouts Check : Constant
  wires:
  RxMsg Process/1 -> Data Store Write/1
  Cast/1 -> Data Store Write5/1  "Vote_s"
  Equal/1 -> Switch6/2
  Data Store Read/1 -> Ensure no self votes or failed master reelected2/2(Sync Timeout), Ensure no self votes or failed master reelected1/2(Sync Timeout), Ensure no self votes or failed master reelected/2(Sync Timeout), Switch5/2
  Switch5/1 -> Cast/1
  Switch6/1 -> Switch5/3
  Data Store Read21/1 -> Switch5/1
  Ensure no self votes or failed master reelected2/1(Out1) -> Max/3
  Constant5/1 -> Switch7/1
  Ensure no self votes or failed master reelected1/1(Out1) -> Max/2, Equal5/2
  Constant4/1 -> Switch6/1
  Constant6/1 -> Switch7/3
  Switch7/1 -> Switch6/3
  Constant1/1 -> Ensure no self votes or failed master reelected1/1(Node ID)
  Constant2/1 -> Ensure no self votes or failed master reelected2/1(Node ID)
  Data Store Read1/1 -> Ensure no self votes or failed master reelected/3(Error counter)
  Equal5/1 -> Switch7/2
  Constant/1 -> Ensure no self votes or failed master reelected/1(Node ID)
  Max/1 -> Equal/2, Equal5/1
  Ensure no self votes or failed master reelected/1(Out1) -> Equal/1, Max/1
  Data Store Read2/1 -> Ensure no self votes or failed master reelected1/3(Error counter)
  Data Store Read3/1 -> Ensure no self votes or failed master reelected2/3(Error counter)
  Timeouts Check/1 -> Data Store Write1/1

== system HANcoder_E407_GTSync_v3_clean/HANcoder STM32 Target - E407-STM32 algorithm/Global Ticks Increment/CAN Management/Matrix Cycle Manager/Vote1 Msg ==
  note: Reception ID
      |    Sync Msg: 1
      |    Vote Node 1: 12
      |    Vote Node 2: 22
      |    Vote Node 3: 32
  note: Message Information
      |    Sync: BoardID
      |    Vote: Vote information
  note: Transmission ID
      |    Sync Msg: 1
      |    Vote Node 1: 12
      |    Vote Node 2: 22
      |    Vote Node 3: 32
  note: Message Data
      |    Every message sends
      |    Local_Time as Data
  note: Basic Cycle 0
      | Time Window 1
      | Message Sent: < Only if BoardID == 1 >
      | 	TxMessage ID: Vote1
      | 	Message Header: Vote
      | 	Message buffert : Local Time
      | Message Receive: < Only if BoardID ~= 1 >
      | 	RxMessage ID: Vote1
  note: Send Message condition
  note: Next State
  note: Message Data (2)
      |    Basic cycle for Sync
  Enable : EnablePort
  Cast : DataTypeConversion  OutDataTypeStr=uint32
  Cast1 : DataTypeConversion  OutDataTypeStr=uint32
  Cast3 : DataTypeConversion  OutDataTypeStr=uint32
  Cast4 : DataTypeConversion  OutDataTypeStr=uint8
  Constant : Constant  Value=Vote1_ID
  Constant1 : Constant
  Constant18 : Constant  Value=comm_delay_estimation
  Constant2 : Constant  Value=Vote1_ID
  Data Store Read : DataStoreRead  DataStoreName=local_ticks_mem_IRQ
  Data Store Read1 : DataStoreRead  DataStoreName=Board_ID
  Data Store Read2 : DataStoreRead  DataStoreName=Vote
  Data Store Read3 : DataStoreRead  DataStoreName=basic_cycle_count
  Data Store Write : DataStoreWrite  DataStoreName=TW1_State
  Data Store Write1 : DataStoreWrite  DataStoreName=message_buffer_2
  Data Store Write5 : DataStoreWrite  DataStoreName=message_header_buffer
  Data Store Write6 : DataStoreWrite  DataStoreName=RxID_message_buffer
  Data Store Write8 : DataStoreWrite  DataStoreName=TxID_message_buffer
  Data Store Write9 : DataStoreWrite  DataStoreName=message_buffer
  Equal : RelationalOperator  Operator===  OutDataTypeStr=boolean  RndMeth=Simplest
  Minus1 : Sum
  TW1 Finished : Constant  Value=3
  Send_Message_Flag : Outport  OutputWhenDisabled=reset  InitialOutput=0
  wires:
  Constant2/1 -> Cast3/1
  Cast3/1 -> Data Store Write6/1
  Data Store Read2/1 -> Data Store Write5/1
  Constant1/1 -> Equal/2
  Equal/1 -> Send_Message_Flag/1
  Data Store Read1/1 -> Equal/1
  Constant/1 -> Cast/1
  Data Store Read/1 -> Minus1/1
  Cast/1 -> Data Store Write8/1
  Cast1/1 -> Data Store Write9/1
  Minus1/1 -> Cast1/1
  Constant18/1 -> Minus1/2
  TW1 Finished/1 -> Data Store Write/1
  Data Store Read3/1 -> Cast4/1
  Cast4/1 -> Data Store Write1/1

== system HANcoder_E407_GTSync_v3_clean/HANcoder STM32 Target - E407-STM32 algorithm/Global Ticks Increment/CAN Management/Matrix Cycle Manager/Vote2 Msg ==
  note: Send Message condition
  note: Basic Cycle 0
      | Time Window 2
      | Message Sent: < Only if BoardID == 2 >
      | 	TxMessage ID: Vote2
      | 	Message Header: Vote
      | 	Message buffert : Local Time
      | Message Receive: < Only if BoardID ~= 2 >
      | 	RxMessage ID: Vote2
  note: Message Data
      |    Every message sends
      |    Local_Time as Data
  note: Transmission ID
      |    Sync Msg: 1
      |    Vote Node 1: 12
      |    Vote Node 2: 22
      |    Vote Node 3: 32
  note: Message Information
      |    Sync: BoardID
      |    Vote: Vote information
  note: Reception ID
      |    Sync Msg: 1
      |    Vote Node 1: 12
      |    Vote Node 2: 22
      |    Vote Node 3: 32
  note: Message Data (2)
      |    Basic cycle for Sync
  Enable : EnablePort
  Cast : DataTypeConversion  OutDataTypeStr=uint32
  Cast1 : DataTypeConversion  OutDataTypeStr=uint32
  Cast3 : DataTypeConversion  OutDataTypeStr=uint32
  Cast4 : DataTypeConversion  OutDataTypeStr=uint8
  Constant : Constant  Value=Vote2_ID
  Constant1 : Constant  Value=2
  Constant18 : Constant  Value=comm_delay_estimation
  Constant2 : Constant  Value=Vote2_ID
  Data Store Read : DataStoreRead  DataStoreName=local_ticks_mem_IRQ
  Data Store Read1 : DataStoreRead  DataStoreName=Board_ID
  Data Store Read2 : DataStoreRead  DataStoreName=Vote
  Data Store Read3 : DataStoreRead  DataStoreName=basic_cycle_count
  Data Store Write1 : DataStoreWrite  DataStoreName=message_buffer_2
  Data Store Write5 : DataStoreWrite  DataStoreName=message_header_buffer
  Data Store Write6 : DataStoreWrite  DataStoreName=RxID_message_buffer
  Data Store Write8 : DataStoreWrite  DataStoreName=TxID_message_buffer
  Data Store Write9 : DataStoreWrite  DataStoreName=message_buffer
  Equal : RelationalOperator  Operator===  OutDataTypeStr=boolean  RndMeth=Simplest
  Minus1 : Sum
  Send_Message_Flag : Outport  OutputWhenDisabled=reset  InitialOutput=0
  wires:
  Constant18/1 -> Minus1/2
  Minus1/1 -> Cast1/1
  Cast1/1 -> Data Store Write9/1
  Cast/1 -> Data Store Write8/1
  Data Store Read/1 -> Minus1/1
  Constant/1 -> Cast/1
  Data Store Read1/1 -> Equal/1
  Equal/1 -> Send_Message_Flag/1
  Constant1/1 -> Equal/2
  Data Store Read2/1 -> Data Store Write5/1
  Cast3/1 -> Data Store Write6/1
  Constant2/1 -> Cast3/1
  Data Store Read3/1 -> Cast4/1
  Cast4/1 -> Data Store Write1/1

== system HANcoder_E407_GTSync_v3_clean/HANcoder STM32 Target - E407-STM32 algorithm/Global Ticks Increment/CAN Management/Matrix Cycle Manager/Vote3 Msg ==
  note: Reception ID
      |    Sync Msg: 1
      |    Vote Node 1: 12
      |    Vote Node 2: 22
      |    Vote Node 3: 32
  note: Message Information
      |    Sync: BoardID
      |    Vote: Vote information
  note: Transmission ID
      |    Sync Msg: 1
      |    Vote Node 1: 12
      |    Vote Node 2: 22
      |    Vote Node 3: 32
  note: Message Data
      |    Every message sends
      |    Local_Time as Data
  note: Basic Cycle 0
      | Time Window 3
      | Message Sent: < Only if BoardID == 3 >
      | 	TxMessage ID: Vote3
      | 	Message Header: Vote
      | 	Message buffert : Local Time
      | Message Receive: < Only if BoardID ~= 3 >
      | 	RxMessage ID: Vote3
  note: Send Message condition
  note: Message Data (2)
      |    Basic cycle for Sync
  Enable : EnablePort
  Cast : DataTypeConversion  OutDataTypeStr=uint32
  Cast1 : DataTypeConversion  OutDataTypeStr=uint32
  Cast3 : DataTypeConversion  OutDataTypeStr=uint32
  Cast4 : DataTypeConversion  OutDataTypeStr=uint8
  Constant : Constant  Value=Vote3_ID
  Constant1 : Constant  Value=3
  Constant18 : Constant  Value=comm_delay_estimation
  Constant2 : Constant  Value=Vote3_ID
  Data Store Read : DataStoreRead  DataStoreName=local_ticks_mem_IRQ
  Data Store Read1 : DataStoreRead  DataStoreName=Board_ID
  Data Store Read2 : DataStoreRead  DataStoreName=Vote
  Data Store Read3 : DataStoreRead  DataStoreName=basic_cycle_count
  Data Store Write1 : DataStoreWrite  DataStoreName=message_buffer_2
  Data Store Write5 : DataStoreWrite  DataStoreName=message_header_buffer
  Data Store Write6 : DataStoreWrite  DataStoreName=RxID_message_buffer
  Data Store Write8 : DataStoreWrite  DataStoreName=TxID_message_buffer
  Data Store Write9 : DataStoreWrite  DataStoreName=message_buffer
  Equal : RelationalOperator  Operator===  OutDataTypeStr=boolean  RndMeth=Simplest
  Minus1 : Sum
  Send_Message_Flag : Outport  OutputWhenDisabled=reset  InitialOutput=0
  wires:
  Constant2/1 -> Cast3/1
  Cast3/1 -> Data Store Write6/1
  Data Store Read2/1 -> Data Store Write5/1
  Constant1/1 -> Equal/2
  Equal/1 -> Send_Message_Flag/1
  Data Store Read1/1 -> Equal/1
  Constant/1 -> Cast/1
  Data Store Read/1 -> Minus1/1
  Cast/1 -> Data Store Write8/1
  Cast1/1 -> Data Store Write9/1
  Minus1/1 -> Cast1/1
  Constant18/1 -> Minus1/2
  Data Store Read3/1 -> Cast4/1
  Cast4/1 -> Data Store Write1/1

== system HANcoder_E407_GTSync_v3_clean/HANcoder STM32 Target - E407-STM32 algorithm/Global Ticks Increment/CAN Management/CAN Recieve/CAN Receive System/Initialize message reception ==
  note: Initialize CAN policy -----------------------------------------
      |
      | When receiving a message with certain ID, the
      | last message sent with that RX_ID is processed.
      | However, we would like the system to wait until
      | a new message arrives.
      |
      | If new message starts being 0, then we just have
      | to wait for the new message to arrive. If it is already
      | 1, then we have to wait until the message buffer
      | changes.
  Enable : EnablePort
  Data Store Memory : DataStoreMemory  DataStoreName=Init_CAN_RX_State  ReadBeforeWriteMsg=warning  WriteAfterWriteMsg=warning  WriteAfterReadMsg=warning  InitialValue=1  ShowAdditionalParam=off
  Data Store Memory1 : DataStoreMemory  DataStoreName=Local_Msg_Buffer  ReadBeforeWriteMsg=warning  WriteAfterWriteMsg=warning  WriteAfterReadMsg=warning  ShowAdditionalParam=off  OutDataTypeStr=Bus: msg_buffer_type
  Data Store Write : DataStoreWrite  DataStoreName=Initialization_CAN_flag
  Init_CAN_RX : Subsystem
  wires:
  ? -> ?
  ? -> ?
  Init_CAN_RX/1(Init CAN) -> Data Store Write/1

== system HANcoder_E407_GTSync_v3_clean/HANcoder STM32 Target - E407-STM32 algorithm/Global Ticks Increment/CAN Management/CAN Recieve/CAN Receive System/Subsystem ==
  Enable : EnablePort
  Bus Creator : BusCreator  Inputs=9
  CAN receive : Subsystem  Tag=HANcoder_TARGET_STM32_E407  AncestorBlock=HANcoder_STM32_Target/STM32-E407/CAN/CAN/CAN receive  mask(CAN receive){canBus=CAN 2, outputNumber=8, dataType=uint8, byteOrder=off, tsamp=-1}
      mask prompts: canBus "CAN channel"; outputNumber "Output ports"; dataType "Output datatype"; byteOrder "Byte order: Checked = MSB first, unchecked = LSB first."; tsamp "Sample time"
      mask help:
      | Function
      | ==========
      | Receive the newest message from the specified CAN channel.
      |
      | Parameters
      | ==========
      | CAN channel:             The CAN channel to send the message on.
      | Output ports:             The amount of output ports
      | Output datatype:       The datatype of the output ports
      | Byte order:                 Select MSB or LSB first
      | Sample time:              -1 or divisible by base sample time [seconds]
      |
      | Input
      | ==========
      | Port 1:                       CAN ID(uint32) in hexadecimal ie: hex2dec('0a')
      |
      | Output
      | ==========
      | Port 1:                       Checks for new message(int8)
      | Port 2..9                     Message data
      mask init:
      | sfcn_can_receive_mcb(canBus, outputNumber, dataType, byteOrder)
      settings: MoveFcn=drawLogos
      mask Help: web('sfcn_can_receive.html');
      mask TypeOptions canBus: CAN 1 | CAN 2
      mask TypeOptions dataType: int8 | uint8 | int16 | uint16 | int32 | uint32 | boolean
      mask Display:
      | fprintf('Receive on\nCAN %x', canBus);
      | port_label('output', 1, 'new');
      | port_label('input', 1, 'ID');patch([85 91 91],[8 14 2],[1 0 0]);patch([93 93 99],[14 2 8],[0 0 0.35]);
  Constant : Constant  Value=Sync_ID  OutDataTypeStr=uint32
  Output : Outport
  wires:
  CAN receive/2(Out2) -> Bus Creator/2
  CAN receive/3(Out3) -> Bus Creator/3
  CAN receive/4(Out4) -> Bus Creator/4
  CAN receive/5(Out5) -> Bus Creator/5
  CAN receive/6(Out6) -> Bus Creator/6
  CAN receive/7(Out7) -> Bus Creator/7
  CAN receive/8(Out8) -> Bus Creator/8
  CAN receive/9(Out9) -> Bus Creator/9
  CAN receive/1(Out1) -> Bus Creator/1
  Bus Creator/1 -> Output/1
  Constant/1 -> CAN receive/1(In1)

== system HANcoder_E407_GTSync_v3_clean/HANcoder STM32 Target - E407-STM32 algorithm/Global Ticks Increment/CAN Management/CAN Recieve/CAN Receive System/Subsystem1 ==
  Enable : EnablePort
  Bus Creator : BusCreator  Inputs=9
  CAN receive : Subsystem  Tag=HANcoder_TARGET_STM32_E407  AncestorBlock=HANcoder_STM32_Target/STM32-E407/CAN/CAN/CAN receive  mask(CAN receive){canBus=CAN 2, outputNumber=8, dataType=uint8, byteOrder=off, tsamp=-1}
      mask prompts: canBus "CAN channel"; outputNumber "Output ports"; dataType "Output datatype"; byteOrder "Byte order: Checked = MSB first, unchecked = LSB first."; tsamp "Sample time"
      mask help:
      | Function
      | ==========
      | Receive the newest message from the specified CAN channel.
      |
      | Parameters
      | ==========
      | CAN channel:             The CAN channel to send the message on.
      | Output ports:             The amount of output ports
      | Output datatype:       The datatype of the output ports
      | Byte order:                 Select MSB or LSB first
      | Sample time:              -1 or divisible by base sample time [seconds]
      |
      | Input
      | ==========
      | Port 1:                       CAN ID(uint32) in hexadecimal ie: hex2dec('0a')
      |
      | Output
      | ==========
      | Port 1:                       Checks for new message(int8)
      | Port 2..9                     Message data
      mask init:
      | sfcn_can_receive_mcb(canBus, outputNumber, dataType, byteOrder)
      settings: MoveFcn=drawLogos
      mask Help: web('sfcn_can_receive.html');
      mask TypeOptions canBus: CAN 1 | CAN 2
      mask TypeOptions dataType: int8 | uint8 | int16 | uint16 | int32 | uint32 | boolean
      mask Display:
      | fprintf('Receive on\nCAN %x', canBus);
      | port_label('output', 1, 'new');
      | port_label('input', 1, 'ID');patch([85 91 91],[8 14 2],[1 0 0]);patch([93 93 99],[14 2 8],[0 0 0.35]);
  Constant1 : Constant  Value=Vote1_ID  OutDataTypeStr=uint32
  Output : Outport
  wires:
  Constant1/1 -> CAN receive/1(In1)
  Bus Creator/1 -> Output/1
  CAN receive/1(Out1) -> Bus Creator/1
  CAN receive/9(Out9) -> Bus Creator/9
  CAN receive/8(Out8) -> Bus Creator/8
  CAN receive/7(Out7) -> Bus Creator/7
  CAN receive/6(Out6) -> Bus Creator/6
  CAN receive/5(Out5) -> Bus Creator/5
  CAN receive/4(Out4) -> Bus Creator/4
  CAN receive/3(Out3) -> Bus Creator/3
  CAN receive/2(Out2) -> Bus Creator/2

== system HANcoder_E407_GTSync_v3_clean/HANcoder STM32 Target - E407-STM32 algorithm/Global Ticks Increment/CAN Management/CAN Recieve/CAN Receive System/Subsystem2 ==
  Enable : EnablePort
  Bus Creator : BusCreator  Inputs=9
  CAN receive : Subsystem  Tag=HANcoder_TARGET_STM32_E407  AncestorBlock=HANcoder_STM32_Target/STM32-E407/CAN/CAN/CAN receive  mask(CAN receive){canBus=CAN 2, outputNumber=8, dataType=uint8, byteOrder=off, tsamp=-1}
      mask prompts: canBus "CAN channel"; outputNumber "Output ports"; dataType "Output datatype"; byteOrder "Byte order: Checked = MSB first, unchecked = LSB first."; tsamp "Sample time"
      mask help:
      | Function
      | ==========
      | Receive the newest message from the specified CAN channel.
      |
      | Parameters
      | ==========
      | CAN channel:             The CAN channel to send the message on.
      | Output ports:             The amount of output ports
      | Output datatype:       The datatype of the output ports
      | Byte order:                 Select MSB or LSB first
      | Sample time:              -1 or divisible by base sample time [seconds]
      |
      | Input
      | ==========
      | Port 1:                       CAN ID(uint32) in hexadecimal ie: hex2dec('0a')
      |
      | Output
      | ==========
      | Port 1:                       Checks for new message(int8)
      | Port 2..9                     Message data
      mask init:
      | sfcn_can_receive_mcb(canBus, outputNumber, dataType, byteOrder)
      settings: MoveFcn=drawLogos
      mask Help: web('sfcn_can_receive.html');
      mask TypeOptions canBus: CAN 1 | CAN 2
      mask TypeOptions dataType: int8 | uint8 | int16 | uint16 | int32 | uint32 | boolean
      mask Display:
      | fprintf('Receive on\nCAN %x', canBus);
      | port_label('output', 1, 'new');
      | port_label('input', 1, 'ID');patch([85 91 91],[8 14 2],[1 0 0]);patch([93 93 99],[14 2 8],[0 0 0.35]);
  Constant3 : Constant  Value=Vote2_ID  OutDataTypeStr=uint32
  Output : Outport
  wires:
  CAN receive/2(Out2) -> Bus Creator/2
  CAN receive/3(Out3) -> Bus Creator/3
  CAN receive/4(Out4) -> Bus Creator/4
  CAN receive/5(Out5) -> Bus Creator/5
  CAN receive/6(Out6) -> Bus Creator/6
  CAN receive/7(Out7) -> Bus Creator/7
  CAN receive/8(Out8) -> Bus Creator/8
  CAN receive/9(Out9) -> Bus Creator/9
  CAN receive/1(Out1) -> Bus Creator/1
  Bus Creator/1 -> Output/1
  Constant3/1 -> CAN receive/1(In1)
